simulink model "FFT_Ex2"  (R2025a)
settings: Solver=VariableStepAuto  StartTime=0.0  StopTime=10.0  RelTol=1e-3
undefined symbols (not defined in the file): i, L, None, nsvg1369, xcve1752
libraries: dspobslib x1, dspsrcs4 x1, aieUtilities x1, aieDSP x1, dspxfrm3 x1, vmcUtilities x1
settings Model: Creator=sdegala  LastModifiedBy=robg
settings RTWCC: GPUComputeCapability=3.5

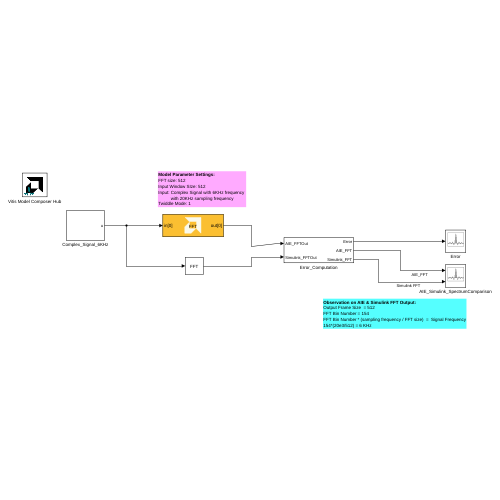
[thumbnail: Simulink's stored preview of the top-level diagram]
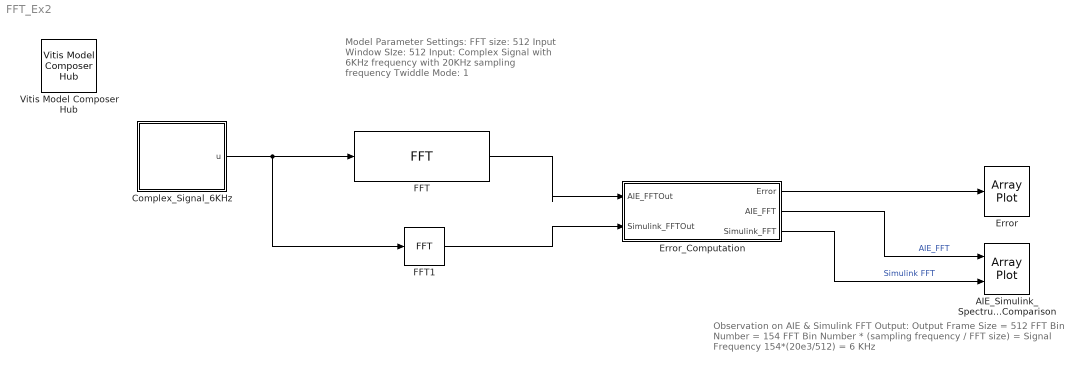
== system FFT_Ex2 ==
  note: Model Parameter Settings:
      | FFT size: 512
      | Input Window SIze: 512
      | Input: Complex Signal with 6KHz frequency
      | with 20KHz sampling frequency
      | Twiddle Mode: 1
  note: Observation on AIE & Simulink FFT Output:
      | Output Frame Size = 512
      | FFT Bin Number = 154
      | FFT Bin Number * (sampling frequency / FFT size) = Signal Frequency
      | 154*(20e3/512) = 6 KHz
  AIE_Simulink_SpectrumComparison : ArrayPlot  NumInputPorts=2  WindowPosition=[83.000000,185.000000,845.000000,423.000000,]  Visible=on  ScopeFrameLocation=window  PlotType=Line  AxesScaling=Manual  YLimits=[-100,1100]  ShowLegend=on
  Complex_Signal_6KHz : Subsystem
  Error : ArrayPlot  WindowPosition=[240.000000,110.000000,800.000000,500.000000,]  Visible=on  ScopeFrameLocation=window
  Error_Computation : Subsystem
  FFT : aieDSP/FFT  AIE_VARIANT=1  data_type=cfloat  data_out_type=cfloat  twiddle_type=cfloat  point_size=512  input_window_size=512  shift_val=0  rnd_mode=Round symmetrical to infinity  sat_mode=0-None  ssr=1  twiddle_mode=1  use_ssr_widget_kernels=off  casc_length=1  transform_fft_nifft=1  TP_API=0  TP_DYN_PT_SIZE=0  blockJsonConstraints=[]  blockJsonConstraintsInternal=[]  spec=vmc_fft.json  SerializedMaskParamNames=[]  SerializedMaskParamValues=[]  SerializedMaskParamVisibilities=[]  block_type=FFT  SerializedMaskParamDataypes=uint|typename|typename|typename|uint|uint|uint|uint|uint|uint|uint|uint|uint|uint|uint|uint  SerializedMaskParamEnumStrArr=0|0|0|0|0|0|0|Round to positive infinity,Round to negative infinity,Round symmetrical to infinity,Round symmetrical to zero,Round convergent to even,Round convergent to odd|0-None,1-Asymmetric,3-Symmetric|0|0|0|0|0|0|0  SerializedMaskParamEnumValArr=0|0|0|0|0|0|0|2,3,4,5,6,7|0,1,3|0|0|0|0|0|0|0  SerializedMaskParamVectorArr=0|0|0|0|0|0|0|0|0|0|0|0|0|0|0|0  SerializedMaskParamKeys=AIE_VARIANT|TT_DATA|TT_OUT_DATA|TT_TWIDDLE|TP_POINT_SIZE|TP_WINDOW_VSIZE|TP_SHIFT|TP_RND|TP_SAT|TP_PARALLEL_POWER|TP_TWIDDLE_MODE|TP_USE_WIDGETS|TP_CASC_LEN|TP_FFT_NIFFT|TP_API|TP_DYN_PT_SIZE
  FFT1 : dspxfrm3/FFT  FFTImplementation=Auto  CompMethod=Table lookup  TableOpt=NEW  TableOptActive=Speed  BitRevOrder=off  Normalize=off  InheritFFTLength=off  FFTLength=512  WrapInput=on  roundingMode=Floor  overflowMode=off  firstCoeffDataTypeStr=Inherit: Same word length as input  firstCoeffLastDataTypeStr=Inherit: Same word length as input  outputMin=[]  outputMax=[]
  Vitis Model Composer Hub : vmcUtilities/Vitis Model Composer Hub  Tag=genX  CodeGeneration=off  CompilationType=HDLCompilation  ExportTypeV2=IP Catalog  StartColumn=1  NumberOfColumns=1  TargetDirectory=./netlist  exportDesign=off  analyzeDesign=off  validateDesignOnHw=off  ExportType=AI Engines  IpVendor=xilinx.com  IpLibrary=hls  IpVersion=1.0  IpHWLanguage=Verilog  AieCompilerOptions={}  AieSimulatorOptions={}  CreateTestbench=off  TestbenchStackSize=10  RunRtlSim=off  RunCSim=off  RunAieSim=off  enableSimulationTimeout=on  enableGraphIterations=on  AieSimTimeout=50000  AieGraphIterations=-1  RunAieSimProfiling=off  LaunchVitisAnalyzer=off  PlotOutput=off  RunX86Sim=off  X86SimTimeout=10  GenHwImage=off  GenLibadfXo=off  GenHwValidationCode=off  PlatformType=Not Specified  HwSystemType=Baremetal  HwValidationTarget=hw  ProjDevice=xcve1752-nsvg1369-1LHP-i-L  ProjDevicePart=xcve1752-nsvg1369-1LHP-i-L  AIEType=AIE  SamplePeriod=-1  ClockFrequency=200  DataPathParallelism=1  xilinxfamily=versalaiedge  part=xcve1752  speed=-1LHP-i-L  package=nsvg1369  directory=./netlist  testbench=off  incr_netlist=off  synthesis_tool=Vivado  clock_wrapper=Clock Enables  dbl_ovrd=According to Block Masks  dcm_input_clock_period=10  sysclk_period=10  simulink_period=1  eval_field=0  LogFileName=''  NThreads=4
  wires:
  FFT/1 -> Error_Computation/1(AIE_FFTOut)
  Error_Computation/2(AIE_FFT) -> AIE_Simulink_SpectrumComparison/1  "AIE_FFT"
  Complex_Signal_6KHz/1(u) -> FFT/1, FFT1/1
  FFT1/1 -> Error_Computation/2(Simulink_FFTOut)
  Error_Computation/1(Error) -> Error/1
  Error_Computation/3(Simulink_FFT) -> AIE_Simulink_SpectrumComparison/2  "Simulink FFT"

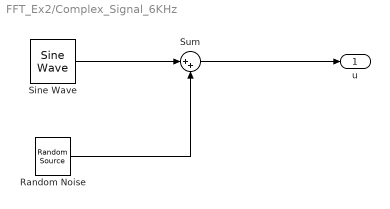
== system FFT_Ex2/Complex_Signal_6KHz ==
  Random Noise : dspobslib/Random Source  SrcType=Gaussian  NormMethod=Ziggurat  CltLength=12  MinVal=0  MaxVal=1  MeanVal=0  VarVal=1e-3  RepMode=Not repeatable  rawSeed=1  IsInherit=off  SampMode=Discrete  SampTime=1/20e3  SampFrame=512  DataType=Single  OutComplex=Real  OutputFrames=off
  Sine Wave : dspsrcs4/Sine Wave  Amplitude=1  Frequency=6e3  Phase=0  SampleMode=Discrete  OutComplex=Complex  CompMethod=Trigonometric fcn  TableSize=Speed  SampleTime=1/20e3  SamplesPerFrame=512  ResetState=Restart at time zero  OutputFrames=off  dataType=single  wordLen=16  udDataType=sfix(16)  fracBitsMode=Best precision  numFracBits=15  OutDataTypeStr=single  LastOutDataTypeStr=single
  Sum : Sum  Inputs=|++
  u : Outport
  wires:
  Sine Wave/1 -> Sum/1
  Sum/1 -> u/1
  Random Noise/1 -> Sum/2

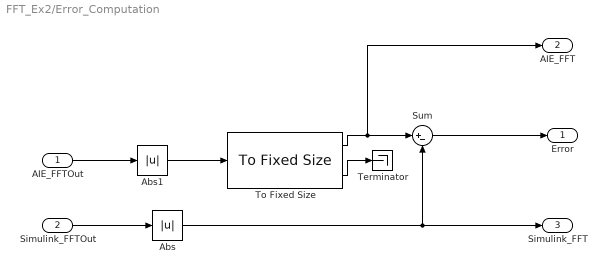
== system FFT_Ex2/Error_Computation ==
  AIE_FFTOut : Inport
  Simulink_FFTOut : Inport  Port=2
  Abs : Abs  SaturateOnIntegerOverflow=off
  Abs1 : Abs  SaturateOnIntegerOverflow=off
  Sum : Sum  Inputs=|+-  AccumDataTypeStr=int32
  Terminator : Terminator
  To Fixed Size : aieUtilities/To Fixed Size  Mode=Produce a valid output signal  OutputSize=512*1  CopyMethod=Buffer samples to form output  HasStatusOutput=on
  Error : Outport
  AIE_FFT : Outport  Port=2
  Simulink_FFT : Outport  Port=3
  wires:
  AIE_FFTOut/1 -> Abs1/1
  Simulink_FFTOut/1 -> Abs/1
  Sum/1 -> Error/1
  Abs1/1 -> To Fixed Size/1
  To Fixed Size/1 -> AIE_FFT/1, Sum/1
  To Fixed Size/2 -> Terminator/1
  Abs/1 -> Simulink_FFT/1, Sum/2
